simulink model "MultirotorModel"  (R2024b)
settings: Solver=VariableStepAuto  StartTime=0.0  StopTime=200  FixedStep=0.005  RelTol=1e-3  EnableMultiTasking=on
undefined symbols (not defined in the file): decyear, Earth, initialConditions, leapyear, Vehicle, WGS84
libraries: sharedutil x2, aerolibatmos2 x1, aerolibgravity2 x1, shared6dof x1, aerolibasang x1, sensorinslib x1, aerolibconvert2 x1, aerolibtransform2 x1
settings Model: DataDictionary=uavPackageDeliveryDataDict.sldd  ModifiedByFormat=The MathWorks, Inc.  Creator=The MathWorks, Inc.  LastModifiedBy=The MathWorks, Inc.
settings SolverCC: AlgebraicLoopSolver=TrustRegion  AutoInsertRateTranBlk=on  MaxZcPerStep=1
settings DataIOCC: LimitDataPoints=on  SaveOutput=off  SaveTime=off  ReturnWorkspaceOutputs=off
settings OptimizationCC: ReuseModelBlockBuffer=off  LifeSpan=inf
settings DebuggingCC: ParameterPrecisionLossMsg=none  UnconnectedInputMsg=warning  UnconnectedOutputMsg=warning  UnconnectedLineMsg=warning  AllowSymbolicDim=off  SFUnexpectedBacktrackingDiag=warning  SFNoUnconditionalDefaultTransitionDiag=warning  SFExecutionAtInitializationDiag=none  ArithmeticOperatorsInVariantConditions=warning
settings ModelReferenceCC: EnableRefExpFcnMdlSchedulingChecks=on  PropagateSignalLabelsOutOfModel=off
settings SFSimCC: SimUseLocalCustomCode=off  CustomCodeUndefinedFunction=UseInterfaceOnly
settings RTWCC: RTWUseLocalCustomCode=off  GPUComputeCapability=3.5  DLArmComputeVersion=19.05
settings CodeAppCC: StateflowObjectComments=on
settings GRTTargetCC: TargetLangStandard=C89/C90 (ANSI)
settings ConfigComp: CovMetricSettings=dw  CovSaveCumulativeToWorkspaceVar=on  CovSaveSingleToWorkspaceVar=on  CovExternalEMLEnable=off

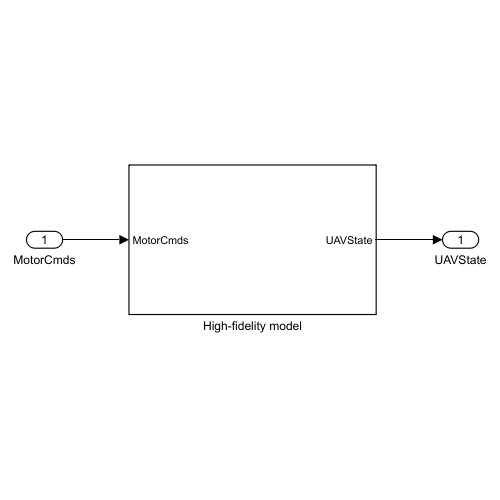
[thumbnail: Simulink's stored preview of the top-level diagram]
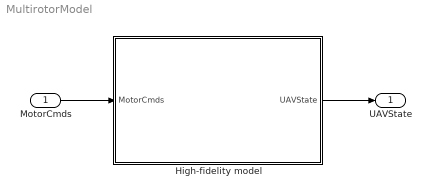
== system MultirotorModel ==
  MotorCmds : Inport
  High-fidelity model : Subsystem
  UAVState : Outport
  wires:
  High-fidelity model/1(UAVState) -> UAVState/1
  MotorCmds/1 -> High-fidelity model/1(MotorCmds)

== system MultirotorModel/High-fidelity model ==
  MotorCmds : Inport
  Environment : Subsystem  TreatAsAtomicUnit=on  VariantControl=VSS_ENVIRONMENT_VARIABLE
  Memory1 : Memory  InheritSampleTime=on  LinearizeMemory=on  LinearizeAsDelay=on
  Plant Model : Subsystem  TreatAsAtomicUnit=on
  UAVState : Outport  OutDataTypeStr=Bus: uavStateBus
  wires:
  MotorCmds/1 -> Plant Model/1(Actuators)
  Environment/1(Environment) -> Plant Model/2(Environment)
  Plant Model/1(UAVState) -> UAVState/1, Memory1/1
  Memory1/1 -> Environment/1(States)

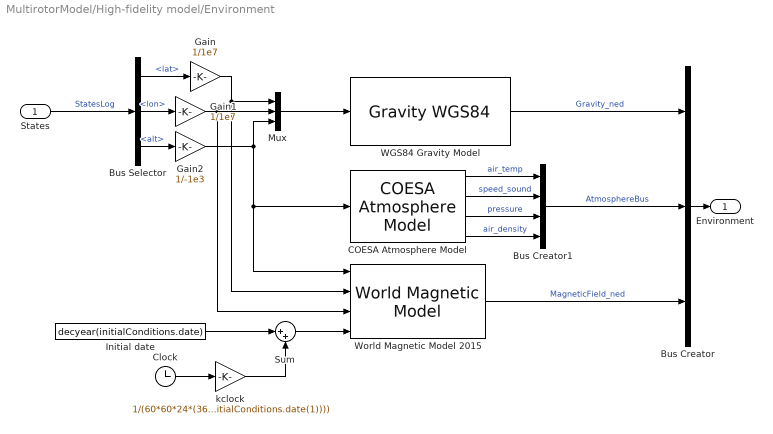
== system MultirotorModel/High-fidelity model/Environment ==
  States : Inport
  Bus Creator : BusCreator  Inputs=3  OutDataTypeStr=Bus: EnvironmentBus  NonVirtualBus=on
  Bus Creator1 : BusCreator  Inputs=4  OutDataTypeStr=Bus: AtmosphereBus  NonVirtualBus=on
  Bus Selector : BusSelector  OutputSignals=gps.lat,gps.lon,gps.alt
  COESA Atmosphere Model : aerolibatmos2/COESA Atmosphere Model  units=Metric (MKS)  spec=1976 COESA-extended U.S. Standard Atmosphere  model=Profile  profile_var=High temperature  profile_percent=1%  profile_alt=5 km (16404 ft)  envelope_var=High temperature  envelope_percent=1%  action=None
  Clock : Clock
  Gain : Gain  Gain=1/1e7  OutDataTypeStr=double
  Gain1 : Gain  Gain=1/1e7  OutDataTypeStr=double
  Gain2 : Gain  Gain=1/-1e3  OutDataTypeStr=double
  Initial date : Constant  Value=decyear(initialConditions.date)
  Mux : Mux  Inputs=3
  Sum : Sum  Inputs=|++
  "WGS84 Gravity Model  " : GravityWGS84  action=None
  World Magnetic Model 2015 : aerolibgravity2/World Magnetic Model  model=WMM2015 V2 (2015-2020)  customFile='WMM2020.COF'  units=Metric (MKS)  time_in=on  month=January  day=1  year=2015  action=Error  h_out=off  dec_out=off  inc_out=off  ti_out=off
  kclock : Gain  Gain=1/(60*60*24*(365 + leapyear(initialConditions.date(1))))
  Environment : Outport  VectorParamsAs1DForOutWhenUnconnected=off
  wires:
  States/1 -> Bus Selector/1  "StatesLog"
  Bus Creator/1 -> Environment/1
  COESA Atmosphere Model/1 -> Bus Creator1/1  "air_temp"
  COESA Atmosphere Model/2 -> Bus Creator1/2  "speed_sound"
  COESA Atmosphere Model/3 -> Bus Creator1/3  "pressure"
  COESA Atmosphere Model/4 -> Bus Creator1/4  "air_density"
  Bus Creator1/1 -> Bus Creator/2  "AtmosphereBus"
  World Magnetic Model 2015/1 -> Bus Creator/3  "MagneticField_ned"
  "WGS84 Gravity Model  "/1 -> Bus Creator/1  "Gravity_ned"
  Clock/1 -> kclock/1
  Initial date/1 -> Sum/1
  Sum/1 -> World Magnetic Model 2015/4
  kclock/1 -> Sum/2
  Mux/1 -> "WGS84 Gravity Model  "/1
  Gain/1 -> World Magnetic Model 2015/2, Mux/1
  Bus Selector/1 -> Gain/1  "<lat>"
  Bus Selector/2 -> Gain1/1  "<lon>"
  Gain1/1 -> World Magnetic Model 2015/3, Mux/2
  Bus Selector/3 -> Gain2/1  "<alt>"
  Gain2/1 -> COESA Atmosphere Model/1, World Magnetic Model 2015/1, Mux/3

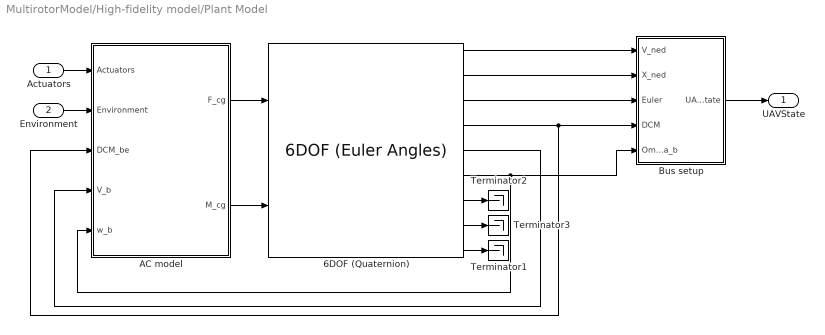
== system MultirotorModel/High-fidelity model/Plant Model ==
  Actuators : Inport
  Environment : Inport  Port=2
  6DOF (Quaternion) : shared6dof/6DOF (Euler Angles)  units=Metric (MKS)  mtype=Fixed  rep=Euler Angles  xme_0=initialConditions.posNED + [0 0 -1]  Vm_0=[0 0 0]  eul_0=[0,0,0]  pm_0=[0,0,0]  mass_0=Vehicle.Airframe.mass  mass_e=0.5  mass_f=2.0  inertia=Vehicle.Airframe.inertia  inertia_e=eye(3)  inertia_f=2*eye(3)  k_quat=Vehicle.SixDOF.quatGain  vre_flag=on  abi_flag=on  aMode=aMode  xme_statename=''  Vm_statename=''  eul_statename=''  quat_statename=''  pm_statename=''  mass_statename=''
  AC model : Subsystem
  Bus setup : Subsystem
  Terminator1 : Terminator
  Terminator2 : Terminator
  Terminator3 : Terminator
  UAVState : Outport  VectorParamsAs1DForOutWhenUnconnected=off
  wires:
  Actuators/1 -> AC model/1(Actuators)
  Environment/1 -> AC model/2(Environment)
  AC model/1(F_cg) -> 6DOF (Quaternion)/1
  AC model/2(M_cg) -> 6DOF (Quaternion)/2
  6DOF (Quaternion)/1 -> Bus setup/1(V_ned)
  6DOF (Quaternion)/2 -> Bus setup/2(X_ned)
  6DOF (Quaternion)/3 -> Bus setup/3(Euler)
  6DOF (Quaternion)/6 -> Bus setup/5(Omega_b), AC model/5(w_b)
  6DOF (Quaternion)/5 -> AC model/4(V_b)
  6DOF (Quaternion)/4 -> Bus setup/4(DCM), AC model/3(DCM_be)
  Bus setup/1(UAVState) -> UAVState/1
  6DOF (Quaternion)/9 -> Terminator1/1
  6DOF (Quaternion)/7 -> Terminator2/1
  6DOF (Quaternion)/8 -> Terminator3/1

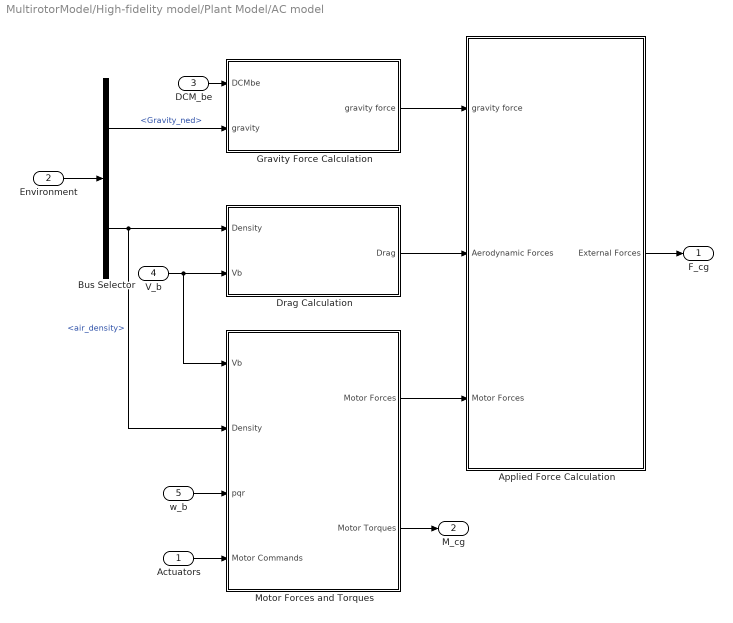
== system MultirotorModel/High-fidelity model/Plant Model/AC model ==
  Actuators : Inport
  Environment : Inport  Port=2
  DCM_be : Inport  Port=3
  V_b : Inport  Port=4  Unit=m/s
  w_b : Inport  Port=5  Unit=rad/s
  Applied Force Calculation : Subsystem
  Bus Selector : BusSelector  OutputSignals=Gravity_ned,AtmosphereBus.air_density
  Drag Calculation : Subsystem
  Gravity Force Calculation : Subsystem
  Motor Forces and Torques : Subsystem
  F_cg : Outport  Unit=N  VectorParamsAs1DForOutWhenUnconnected=off
  M_cg : Outport  Port=2  Unit=N*m  VectorParamsAs1DForOutWhenUnconnected=off
  wires:
  Applied Force Calculation/1(External Forces) -> F_cg/1
  Motor Forces and Torques/2(Motor Torques) -> M_cg/1
  Motor Forces and Torques/1(Motor Forces) -> Applied Force Calculation/3(Motor Forces)
  Bus Selector/1 -> Gravity Force Calculation/2(gravity)  "<Gravity_ned>"
  Gravity Force Calculation/1(gravity force) -> Applied Force Calculation/1(gravity force)
  Environment/1 -> Bus Selector/1
  Bus Selector/2 -> Motor Forces and Torques/2(Density), Drag Calculation/1(Density)  "<air_density>"
  DCM_be/1 -> Gravity Force Calculation/1(DCMbe)
  V_b/1 -> Motor Forces and Torques/1(Vb), Drag Calculation/2(Vb)
  Drag Calculation/1(Drag) -> Applied Force Calculation/2(Aerodynamic Forces)
  Actuators/1 -> Motor Forces and Torques/4(Motor Commands)
  w_b/1 -> Motor Forces and Torques/3(pqr)

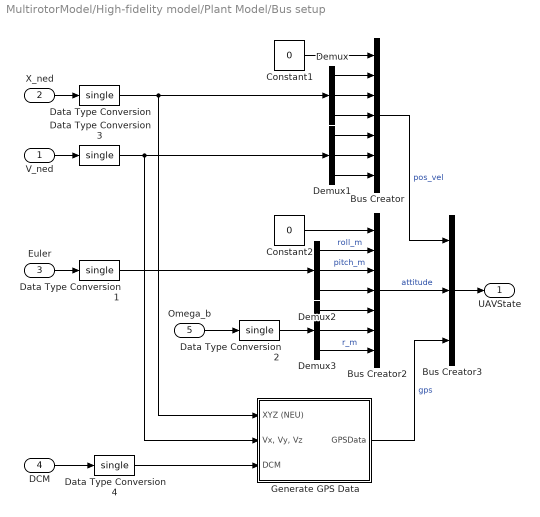
== system MultirotorModel/High-fidelity model/Plant Model/Bus setup ==
  V_ned : Inport  Unit=m/second  PortDimensions=3
  X_ned : Inport  Port=2  Unit=m  PortDimensions=3
  Euler : Inport  Port=3  Unit=rad  PortDimensions=3
  DCM : Inport  Port=4
  Omega_b : Inport  Port=5  Unit=rad/s  PortDimensions=3
  Bus Creator : BusCreator  Inputs=7  OutDataTypeStr=Bus: local_position_ned
      settings: InheritFromInputs=off
  Bus Creator2 : BusCreator  Inputs=7  OutDataTypeStr=Bus: attitudeBus
      settings: InheritFromInputs=off
  Bus Creator3 : BusCreator  Inputs=3  OutDataTypeStr=Bus: uavStateBus
      settings: InheritFromInputs=off
  Constant1 : Constant  Value=0  OutDataTypeStr=uint32
  Constant2 : Constant  Value=0  OutDataTypeStr=uint32
  Data Type Conversion{,1..4} (5 alike) : DataTypeConversion  OutDataTypeStr=single  SaturateOnIntegerOverflow=off  RndMeth=Floor
  Demux{,1..3} (4 alike) : Demux  Outputs=3
  Generate GPS Data : Subsystem
  UAVState : Outport  OutDataTypeStr=Bus: uavStateBus
  wires:
  Demux1/3 -> Bus Creator/7
  Bus Creator3/1 -> UAVState/1
  Demux/2 -> Bus Creator/3
  Demux3/2 -> Bus Creator2/6
  Bus Creator2/1 -> Bus Creator3/2  "attitude"
  Demux1/2 -> Bus Creator/6
  Demux3/1 -> Bus Creator2/5
  Demux/1 -> Bus Creator/2
  Euler/1 -> Data Type Conversion1/1
  Demux2/3 -> Bus Creator2/4
  Demux2/1 -> Bus Creator2/2  "roll_m"
  Bus Creator/1 -> Bus Creator3/1  "pos_vel"
  Constant2/1 -> Bus Creator2/1
  Demux2/2 -> Bus Creator2/3  "pitch_m"
  Demux3/3 -> Bus Creator2/7  "r_m"
  Demux1/1 -> Bus Creator/5
  V_ned/1 -> Data Type Conversion3/1
  Omega_b/1 -> Data Type Conversion2/1
  Demux/3 -> Bus Creator/4
  Constant1/1 -> Bus Creator/1
  Generate GPS Data/1(GPSData) -> Bus Creator3/3  "gps"
  X_ned/1 -> Data Type Conversion/1
  Data Type Conversion/1 -> Generate GPS Data/1(XYZ (NEU)), Demux/1
  Data Type Conversion2/1 -> Demux3/1
  Data Type Conversion1/1 -> Demux2/1
  Data Type Conversion3/1 -> Demux1/1, Generate GPS Data/2("Vx, Vy, Vz")
  DCM/1 -> Data Type Conversion4/1
  Data Type Conversion4/1 -> Generate GPS Data/3(DCM)

== system MultirotorModel/High-fidelity model/Plant Model/AC model/Applied Force Calculation ==
  gravity force : Inport  Unit=N
  Aerodynamic Forces : Inport  Port=2  Unit=N
  Motor Forces : Inport  Port=3  Unit=N
  Add1 : Sum  Inputs=+++
  Signal Specification : SignalSpecification  Dimensions=3
  External Forces : Outport  Unit=N  VectorParamsAs1DForOutWhenUnconnected=off
  wires:
  Add1/1 -> Signal Specification/1
  Motor Forces/1 -> Add1/3  "Motor Thrust"
  Aerodynamic Forces/1 -> Add1/2
  gravity force/1 -> Add1/1
  Signal Specification/1 -> External Forces/1

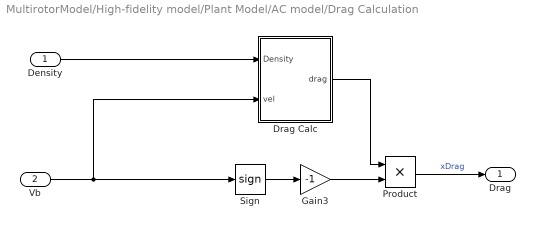
== system MultirotorModel/High-fidelity model/Plant Model/AC model/Drag Calculation ==
  Density : Inport  Unit=kg/m^3
  Vb : Inport  Port=2  Unit=m/second
  Drag Calc : Subsystem
  Gain3 : Gain  Gain=-1
  Product : Product  RndMeth=Zero
  Sign : Signum  ZeroCross=off
  Drag : Outport  Unit=N  VectorParamsAs1DForOutWhenUnconnected=off
  wires:
  Density/1 -> Drag Calc/1(Density)
  Sign/1 -> Gain3/1
  Drag Calc/1(drag) -> Product/1
  Gain3/1 -> Product/2
  Product/1 -> Drag/1  "xDrag"
  Vb/1 -> Sign/1, Drag Calc/2(vel)

== system MultirotorModel/High-fidelity model/Plant Model/AC model/Gravity Force Calculation ==
  DCMbe : Inport
  gravity : Inport  Port=2  Unit=m/s^2
  Gain1 : Gain  Gain=Vehicle.Airframe.mass
  Product : Product  Multiplication=Matrix(*)
  gravity force : Outport  Unit=N  VectorParamsAs1DForOutWhenUnconnected=off
  wires:
  gravity/1 -> Gain1/1
  Gain1/1 -> Product/2  "gravity force NED"
  Product/1 -> gravity force/1
  DCMbe/1 -> Product/1

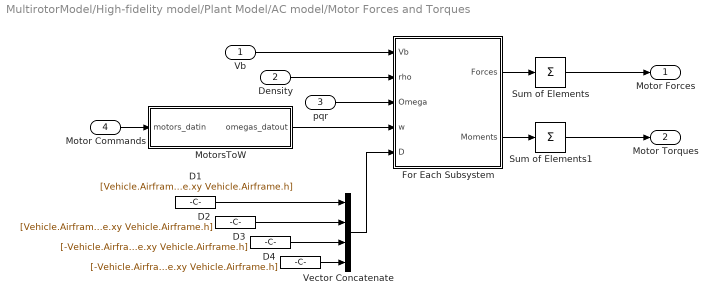
== system MultirotorModel/High-fidelity model/Plant Model/AC model/Motor Forces and Torques ==
  Vb : Inport
  Density : Inport  Port=2
  pqr : Inport  Port=3
  Motor Commands : Inport  Port=4
  D1 : Constant  Value=[Vehicle.Airframe.xy -Vehicle.Airframe.xy Vehicle.Airframe.h]
  D2 : Constant  Value=[Vehicle.Airframe.xy Vehicle.Airframe.xy Vehicle.Airframe.h]
  D3 : Constant  Value=[-Vehicle.Airframe.xy Vehicle.Airframe.xy Vehicle.Airframe.h]
  D4 : Constant  Value=[-Vehicle.Airframe.xy -Vehicle.Airframe.xy Vehicle.Airframe.h]
  For Each Subsystem : Subsystem  TreatAsAtomicUnit=on
  MotorsToW : Subsystem
  Sum of Elements : Sum  Inputs=+  CollapseMode=Specified dimension  CollapseDim=2
  Sum of Elements1 : Sum  Inputs=+  CollapseMode=Specified dimension  CollapseDim=2
  Vector Concatenate : Concatenate  NumInputs=4  Mode=Multidimensional array  ConcatenateDimension=2
  Motor Forces : Outport  Unit=N  VectorParamsAs1DForOutWhenUnconnected=off
  Motor Torques : Outport  Port=2  Unit=N*m  VectorParamsAs1DForOutWhenUnconnected=off
  wires:
  D4/1 -> Vector Concatenate/4
  MotorsToW/1(omegas_datout) -> For Each Subsystem/4(w)
  Vector Concatenate/1 -> For Each Subsystem/5(D)
  For Each Subsystem/2(Moments) -> Sum of Elements1/1
  pqr/1 -> For Each Subsystem/3(Omega)
  Vb/1 -> For Each Subsystem/1(Vb)
  Motor Commands/1 -> MotorsToW/1(motors_datin)
  D1/1 -> Vector Concatenate/1
  D3/1 -> Vector Concatenate/3
  D2/1 -> Vector Concatenate/2
  Sum of Elements1/1 -> Motor Torques/1
  Density/1 -> For Each Subsystem/2(rho)
  Sum of Elements/1 -> Motor Forces/1
  For Each Subsystem/1(Forces) -> Sum of Elements/1

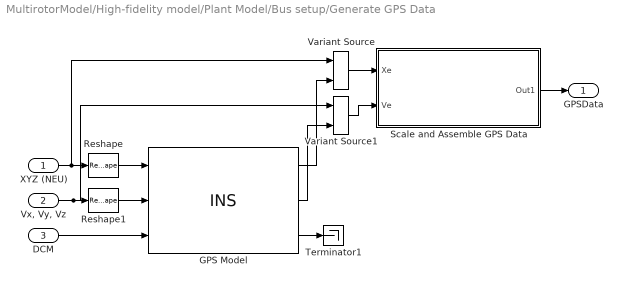
== system MultirotorModel/High-fidelity model/Plant Model/Bus setup/Generate GPS Data ==
  XYZ (NEU) : Inport
  "Vx, Vy, Vz" : Inport  Port=2
  DCM : Inport  Port=3
  GPS Model : sensorinslib/INS  MountingLocation=[0 0 0]  RollAccuracy=0.2  PitchAccuracy=0.2  YawAccuracy=1  PositionAccuracy=0.85  VelocityAccuracy=0.05  UseAccelAndAngVel=off  AccelerationAccuracy=0  AngularVelocityAccuracy=0  TimeInput=off  PositionErrorFactor=[0 0 0]  SeedDouble=67  SimulateUsing=Code generation
  Reshape : Reshape  OutputDimensionality=Customize  OutputDimensions=[1 3]
  Reshape1 : Reshape  OutputDimensionality=Customize  OutputDimensions=[1 3]
  "Scale and Assemble GPS Data " : Subsystem
  Terminator1 : Terminator
  Variant Source : VariantSource  VariantControlMode=label  LabelModeActiveChoice=Model
  Variant Source1 : VariantSource  VariantControlMode=label  LabelModeActiveChoice=Model
  GPSData : Outport  VectorParamsAs1DForOutWhenUnconnected=off
  wires:
  DCM/1 -> GPS Model/3
  "Vx, Vy, Vz"/1 -> Variant Source1/1, Reshape1/1
  XYZ (NEU)/1 -> Variant Source/1, Reshape/1
  GPS Model/3 -> Terminator1/1
  Reshape/1 -> GPS Model/1
  Reshape1/1 -> GPS Model/2
  "Scale and Assemble GPS Data "/1(Out1) -> GPSData/1
  GPS Model/1 -> Variant Source/2
  Variant Source1/1 -> "Scale and Assemble GPS Data "/2(Ve)
  GPS Model/2 -> Variant Source1/2
  Variant Source/1 -> "Scale and Assemble GPS Data "/1(Xe)

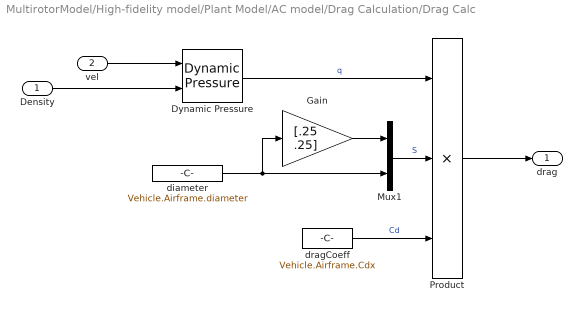
== system MultirotorModel/High-fidelity model/Plant Model/AC model/Drag Calculation/Drag Calc ==
  Density : Inport  Unit=kg/m^3
  vel : Inport  Port=2  Unit=m/s
  Dynamic Pressure : aerolibasang/Dynamic Pressure
  Gain : Gain  Gain=[.25 .25]
  Mux1 : Mux  Inputs=2
  Product : Product  Inputs=3  RndMeth=Zero
  diameter : Constant  Value=Vehicle.Airframe.diameter  SampleTime=0
  dragCoeff : Constant  Value=Vehicle.Airframe.Cdx  SampleTime=0
  drag : Outport  Unit=N  VectorParamsAs1DForOutWhenUnconnected=off
  wires:
  Product/1 -> drag/1
  dragCoeff/1 -> Product/3  "Cd"
  Dynamic Pressure/1 -> Product/1  "q"
  diameter/1 -> Gain/1, Mux1/2
  Mux1/1 -> Product/2  "S"
  Gain/1 -> Mux1/1
  vel/1 -> Dynamic Pressure/1
  Density/1 -> Dynamic Pressure/2

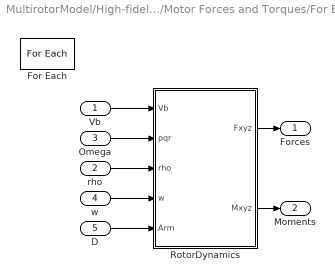
== system MultirotorModel/High-fidelity model/Plant Model/AC model/Motor Forces and Torques/For Each Subsystem ==
  Vb : Inport  PortDimensions=3
  rho : Inport  Port=2  PortDimensions=1
  Omega : Inport  Port=3
  w : Inport  Port=4  Partition=on  PartitionDimension=2  PartitionWidth=1  PartitionOffset=0
  D : Inport  Port=5  Partition=on  PartitionDimension=2  PartitionWidth=1  PartitionOffset=0
  For Each : ForEach  DisableCoverage=on
  RotorDynamics : Subsystem  TreatAsAtomicUnit=on
      mask init:
      | aeroicon('aeroblk');
      settings: RTWFcnNameOpts=Use subsystem name  RTWFileNameOpts=Use function name
  Forces : Outport  ConcatenationDimension=2  VectorParamsAs1DForOutWhenUnconnected=off
  Moments : Outport  Port=2  ConcatenationDimension=2  VectorParamsAs1DForOutWhenUnconnected=off
  wires:
  RotorDynamics/1(Fxyz) -> Forces/1
  RotorDynamics/2(Mxyz) -> Moments/1
  Vb/1 -> RotorDynamics/1(Vb)
  Omega/1 -> RotorDynamics/2(pqr)
  rho/1 -> RotorDynamics/3(rho)
  D/1 -> RotorDynamics/5(Arm)
  w/1 -> RotorDynamics/4(w)

== system MultirotorModel/High-fidelity model/Plant Model/AC model/Motor Forces and Torques/MotorsToW ==
  motors_datin : Inport
  Motordirections : Gain  Gain=[1 -1 1 -1]  ParamDataTypeStr=single  OutDataTypeStr=Inherit: Inherit via back propagation  SaturateOnIntegerOverflow=on
  Motordirections1 : Gain  Gain=[1 -1 1 -1]  ParamDataTypeStr=single  OutDataTypeStr=Inherit: Inherit via back propagation  SaturateOnIntegerOverflow=on
  Saturation5 : Saturate  UpperLimit=Vehicle.Motor.maxLimit  LowerLimit=Vehicle.Motor.minLimit  OutDataTypeStr=Inherit: Inherit via back propagation
  Signed Sqrt : Sqrt  Operator=signedSqrt  OutDataTypeStr=Inherit: Inherit via back propagation
  motorsToW2_Gain : Gain  Gain=Vehicle.Motor.commandToW2Gain  ParamDataTypeStr=single  OutDataTypeStr=Inherit: Inherit via back propagation  SaturateOnIntegerOverflow=on
  omegas_datout : Outport  VectorParamsAs1DForOutWhenUnconnected=off
  wires:
  motorsToW2_Gain/1 -> Signed Sqrt/1
  Motordirections/1 -> Saturation5/1
  Saturation5/1 -> Motordirections1/1
  Motordirections1/1 -> motorsToW2_Gain/1
  Signed Sqrt/1 -> omegas_datout/1
  motors_datin/1 -> Motordirections/1

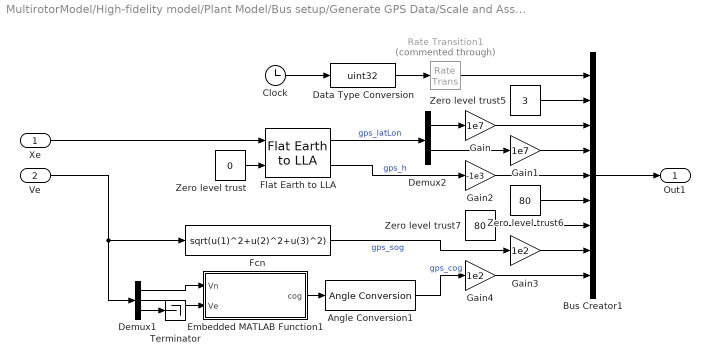
== system MultirotorModel/High-fidelity model/Plant Model/Bus setup/Generate GPS Data/Scale and Assemble GPS Data  ==
  Xe : Inport
  Ve : Inport  Port=2
  Angle Conversion1 : aerolibconvert2/Angle Conversion  IU=rad  OU=deg
  Bus Creator1 : BusCreator  Inputs=9  OutDataTypeStr=Bus: gps_raw_int  NonVirtualBus=on
      settings: InheritFromInputs=off
  Clock : Clock
      settings: AttributesFormatString=Decimation: %<Decimation>
  Data Type Conversion : DataTypeConversion  OutDataTypeStr=uint32  SaturateOnIntegerOverflow=off  RndMeth=Floor
  Demux1 : Demux  Outputs=3
  Demux2 : Demux  Outputs=2
  Embedded MATLAB Function1 : MATLAB Function  TreatAsAtomicUnit=on
  Fcn : Fcn  Expr=sqrt(u(1)^2+u(2)^2+u(3)^2)
  Flat Earth to LLA : aerolibtransform2/Flat Earth to LLA  units=Metric (MKS)  ptype=Earth (WGS84)  F=1/298.257223563  R=6378137  refPosPort=off  LL0=uavIC_latLon  psi=0
  Gain : Gain  Gain=1e7  OutDataTypeStr=int32
  Gain1 : Gain  Gain=1e7  OutDataTypeStr=int32
  Gain2 : Gain  Gain=-1e3  OutDataTypeStr=int32
  Gain3 : Gain  Gain=1e2  OutDataTypeStr=uint16
  Gain4 : Gain  Gain=1e2  OutDataTypeStr=uint16
  Rate Transition1 : RateTransition  Commented=through  OutPortSampleTime=0.005
  Terminator : Terminator
  Zero level trust : Constant  Value=0
      settings: AttributesFormatString=%<Value>
  Zero level trust5 : Constant  Value=3  OutDataTypeStr=uint8
      settings: AttributesFormatString=%<Value>
  Zero level trust6 : Constant  Value=80  OutDataTypeStr=uint16
      settings: AttributesFormatString=%<Value>
  Zero level trust7 : Constant  Value=80  OutDataTypeStr=uint16
      settings: AttributesFormatString=%<Value>
  Out1 : Outport
  wires:
  Demux2/1 -> Gain/1
  Gain/1 -> Bus Creator1/3
  Gain4/1 -> Bus Creator1/9
  Demux2/2 -> Gain1/1
  Embedded MATLAB Function1/1(cog) -> Angle Conversion1/1
  Rate Transition1/1 -> Bus Creator1/1
  Zero level trust6/1 -> Bus Creator1/6
  Gain3/1 -> Bus Creator1/8
  Clock/1 -> Data Type Conversion/1
  Ve/1 -> Demux1/1, Fcn/1
  Zero level trust7/1 -> Bus Creator1/7
  Data Type Conversion/1 -> Rate Transition1/1
  Demux1/2 -> Embedded MATLAB Function1/2(Ve)
  Zero level trust5/1 -> Bus Creator1/2
  Demux1/1 -> Embedded MATLAB Function1/1(Vn)
  Flat Earth to LLA/1 -> Demux2/1  "gps_latLon"
  Gain2/1 -> Bus Creator1/5
  Fcn/1 -> Gain3/1  "gps_sog"
  Gain1/1 -> Bus Creator1/4
  Flat Earth to LLA/2 -> Gain2/1  "gps_h"
  Zero level trust/1 -> Flat Earth to LLA/2
  Angle Conversion1/1 -> Gain4/1  "gps_cog"
  Demux1/3 -> Terminator/1
  Xe/1 -> Flat Earth to LLA/1
  Bus Creator1/1 -> Out1/1

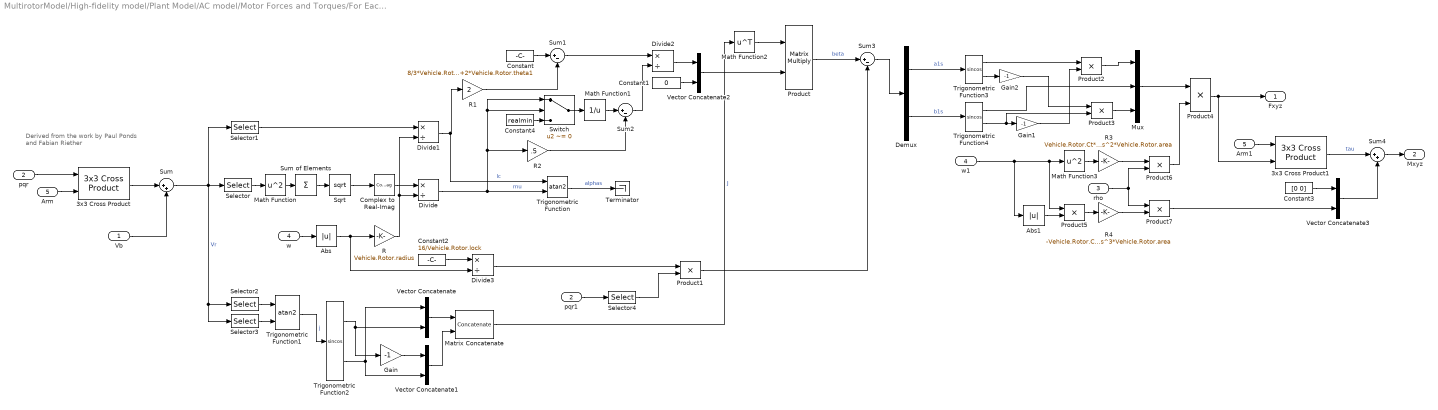
== system MultirotorModel/High-fidelity model/Plant Model/AC model/Motor Forces and Torques/For Each Subsystem/RotorDynamics ==
  note: Derived from the work by Paul Ponds
      | and Fabian Riether
  Vb : Inport  PortDimensions=3
  pqr : Inport  Port=2  PortDimensions=3
  rho : Inport  Port=3  PortDimensions=1
  w : Inport  Port=4  PortDimensions=[1 1]
  Arm : Inport  Port=5  PortDimensions=[3 1]
  3x3 Cross Product : sharedutil/3x3 Cross Product  aMode=aMode
  3x3 Cross Product1 : sharedutil/3x3 Cross Product  aMode=aMode
  Abs : Abs  SaturateOnIntegerOverflow=off
  Abs1 : Abs  SaturateOnIntegerOverflow=off
  Arm1 : InportShadow  Port=5  PortDimensions=[3 1]
  Complex to Real-Imag : ComplexToRealImag  Output=Real
  Constant : Constant  Value=8/3*Vehicle.Rotor.theta0+2*Vehicle.Rotor.theta1
  Constant1 : Constant  Value=0
  Constant2 : Constant  Value=16/Vehicle.Rotor.lock
  Constant3 : Constant  Value=[0 0]
  Constant4 : Constant  Value=realmin
  Demux : Demux  Outputs=2
  Divide{,1..3} (4 alike) : Product  Inputs=*/
  Gain : Gain  Gain=-1
  Gain1 : Gain  Gain=-1
  Gain2 : Gain  Gain=-1
  Math Function : Math  Operator=square  SignedPower=on
  Math Function1 : Math  Operator=reciprocal  SignedPower=on
  Math Function2 : Math  Operator=transpose  SignedPower=on
  Math Function3 : Math  Operator=square  SignedPower=on
  Matrix Concatenate : Concatenate  Mode=Multidimensional array  ConcatenateDimension=2
  Mux : Mux  Inputs=3
  Product : Product  Multiplication=Matrix(*)
  Product{1..7} (7 alike) : Product
  R : Gain  Gain=Vehicle.Rotor.radius
  R1 : Gain  Gain=2
  R2 : Gain  Gain=.5
  R3 : Gain  Gain=Vehicle.Rotor.Ct*Vehicle.Rotor.radius^2*Vehicle.Rotor.area
  R4 : Gain  Gain=-Vehicle.Rotor.Cq*Vehicle.Rotor.radius^3*Vehicle.Rotor.area
  Selector : Selector  InputPortWidth=3  IndexOptions=Index vector (dialog)  Indices=[1 2]  OutputSizes=1
  Selector1 : Selector  InputPortWidth=3  IndexOptions=Index vector (dialog)  Indices=[3]  OutputSizes=1
  Selector2 : Selector  InputPortWidth=3  IndexOptions=Index vector (dialog)  Indices=[2]  OutputSizes=1
  Selector3 : Selector  InputPortWidth=3  IndexOptions=Index vector (dialog)  Indices=[1]  OutputSizes=1
  Selector4 : Selector  InputPortWidth=3  IndexOptions=Index vector (dialog)  Indices=[2 1]  OutputSizes=1
  Sqrt : Sqrt  OutputSignalType=complex
  Sum : Sum  Inputs=|++
  Sum of Elements : Sum  Inputs=+
  Sum1 : Sum  Inputs=|+-
  Sum2 : Sum  Inputs=|+-
  Sum3 : Sum  Inputs=|+-
  Sum4 : Sum  Inputs=|++
  Switch : Switch  Criteria=u2 ~= 0  SaturateOnIntegerOverflow=off  InputSameDT=off
  Terminator : Terminator
  Trigonometric Function : Trigonometry  Operator=atan2
  Trigonometric Function1 : Trigonometry  Operator=atan2
  Trigonometric Function2 : Trigonometry  Operator=sincos
  Trigonometric Function3 : Trigonometry  Operator=sincos
  Trigonometric Function4 : Trigonometry  Operator=sincos
  Vector Concatenate{,1..3} (4 alike) : Concatenate
  pqr1 : InportShadow  Port=2  PortDimensions=3
  w1 : InportShadow  Port=4  PortDimensions=[1 1]
  Fxyz : Outport  PortDimensions=[3 1]  VectorParamsAs1DForOutWhenUnconnected=off
  Mxyz : Outport  Port=2  PortDimensions=[3 1]  VectorParamsAs1DForOutWhenUnconnected=off
  wires:
  Complex to Real-Imag/1 -> Divide/1
  Sqrt/1 -> Complex to Real-Imag/1
  Constant4/1 -> Switch/3
  Switch/1 -> Math Function1/1
  Product1/1 -> Sum3/2
  rho/1 -> Product7/1, Product6/2
  Product7/1 -> Vector Concatenate3/2
  Product6/1 -> Product4/2
  Sum4/1 -> Mxyz/1
  3x3 Cross Product1/1 -> Sum4/1  "tau"
  Product4/1 -> Fxyz/1, 3x3 Cross Product1/2
  Arm1/1 -> 3x3 Cross Product1/1
  Vector Concatenate3/1 -> Sum4/2
  Constant3/1 -> Vector Concatenate3/1
  R4/1 -> Product7/2
  Product5/1 -> R4/1
  Abs1/1 -> Product5/2
  R3/1 -> Product6/1
  Mux/1 -> Product4/1
  Gain2/1 -> Product3/1
  Product3/1 -> Mux/3
  Trigonometric Function3/2 -> Gain2/1
  Trigonometric Function4/1 -> Mux/2
  Product2/1 -> Mux/1
  Trigonometric Function3/1 -> Product2/1
  Gain1/1 -> Product2/2
  Trigonometric Function4/2 -> Gain1/1, Product3/2
  Demux/2 -> Trigonometric Function4/1  "b1s"
  Demux/1 -> Trigonometric Function3/1  "a1s"
  Sum3/1 -> Demux/1
  Math Function3/1 -> R3/1
  w1/1 -> Math Function3/1, Product5/1, Abs1/1
  Divide3/1 -> Product1/1
  Abs/1 -> R/1, Divide3/2
  Selector4/1 -> Product1/2
  pqr1/1 -> Selector4/1
  Constant2/1 -> Divide3/1
  Product/1 -> Sum3/1  "beta"
  Math Function2/1 -> Product/1
  Vector Concatenate2/1 -> Product/2
  Constant1/1 -> Vector Concatenate2/2
  Divide2/1 -> Vector Concatenate2/1
  Sum2/1 -> Divide2/2
  R2/1 -> Sum2/2
  Math Function1/1 -> Sum2/1
  Sum1/1 -> Divide2/1
  R1/1 -> Sum1/2
  Constant/1 -> Sum1/1
  Matrix Concatenate/1 -> Math Function2/1  "J"
  Vector Concatenate1/1 -> Matrix Concatenate/2
  Vector Concatenate/1 -> Matrix Concatenate/1
  Trigonometric Function2/1 -> Gain/1, Vector Concatenate/2
  Gain/1 -> Vector Concatenate1/1
  Trigonometric Function2/2 -> Vector Concatenate/1, Vector Concatenate1/2
  Trigonometric Function1/1 -> Trigonometric Function2/1  "j"
  Selector3/1 -> Trigonometric Function1/2
  Selector2/1 -> Trigonometric Function1/1
  Trigonometric Function/1 -> Terminator/1  "alphas"
  Divide1/1 -> Trigonometric Function/1, R1/1  "lc"
  Selector1/1 -> Divide1/1
  Divide/1 -> Trigonometric Function/2, Switch/1, Switch/2, R2/1  "mu"
  R/1 -> Divide/2, Divide1/2
  w/1 -> Abs/1
  Arm/1 -> 3x3 Cross Product/2
  pqr/1 -> 3x3 Cross Product/1
  Sum of Elements/1 -> Sqrt/1
  Math Function/1 -> Sum of Elements/1
  Selector/1 -> Math Function/1
  Sum/1 -> Selector/1, Selector1/1, Selector2/1, Selector3/1  "Vr"
  Vb/1 -> Sum/2
  3x3 Cross Product/1 -> Sum/1

== matlab function MultirotorModel/High-fidelity model/Plant Model/Bus setup/Generate GPS Data/Scale and Assemble GPS Data /Embedded MATLAB Function1 ==
  data: cog output; Vn input; Ve input
function cog = getCOG(Vn, Ve)
% This block supports an embeddable subset of the MATLAB language.
% See the help menu for details. 

cog = atan2(Ve,Vn);
if cog < 0;
    cog = cog + 2*pi;
end
